simulink model "ulrich2017"  (R2023a)
settings: Solver=ode4  StartTime=0.0  StopTime=tsim  FixedStep=baseRate  RelTol=1e-6  AbsTol=1e-6
values from neighbouring files (symbols this model uses):
  Gamma1_el = 0.12    [initSpotDefaultParam.m]
  Gamma1_sh = 0.005    [initSpotDefaultParam.m]
  Gamma1_wr = 0.025    [initSpotDefaultParam.m]
  Gamma2_el = 5    [initSpotDefaultParam.m]
  Gamma2_sh = 5    [initSpotDefaultParam.m]
  Gamma2_wr = 5    [initSpotDefaultParam.m]
  Gamma3_el = 10    [initSpotDefaultParam.m]
  Gamma3_sh = 40    [initSpotDefaultParam.m]
  Gamma3_wr = 40    [initSpotDefaultParam.m]
  Gamma4_el = 0.039    [initSpotDefaultParam.m]
  Gamma4_sh = 0.015    [initSpotDefaultParam.m]
  Gamma4_wr = 0.029    [initSpotDefaultParam.m]
  Gamma5_el = 800    [initSpotDefaultParam.m]
  Gamma5_sh = 800    [initSpotDefaultParam.m]
  Gamma5_wr = 800    [initSpotDefaultParam.m]
  Gamma6_el = 0.000001    (= 1e-06)    [initSpotDefaultParam.m]
  Gamma6_sh = 0.005    [initSpotDefaultParam.m]
  Gamma6_wr = 0.02    [initSpotDefaultParam.m]
  Kd_elarm = 0.8    [initSpotDefaultParam.m]
  Kd_sharm = 1.0    (= 1)    [initSpotDefaultParam.m]
  Kd_wrarm = 0.6    [initSpotDefaultParam.m]
  Kp_elarm = 1.2    [initSpotDefaultParam.m]
  Kp_sharm = 1.5    [initSpotDefaultParam.m]
  Kp_wrarm = 2    [initSpotDefaultParam.m]
  PWMFreq = 5    [initSpotDefaultParam.m]
  Tz_lim_elarm = .1    (= 0.1)    [initSpotDefaultParam.m]
  Tz_lim_sharm = .1    (= 0.1)    [initSpotDefaultParam.m]
  Tz_lim_wrarm = .1    (= 0.1)    [initSpotDefaultParam.m]
undefined symbols (not defined in the file or in its folder): a1, a2, a3, b0, b1, b2, b3, baseRate, DiscIntNeverNeededParam, drop_states_ARM, drop_states_BLACK, drop_states_BLUE, drop_states_RED, F_Black_X_nominal, F_Black_Y_nominal, F_Blue_X_nominal, F_Blue_Y_nominal, F_red_X_nominal, F_red_Y_nominal, F_thrusters_BLACK, F_thrusters_BLUE, F_thrusters_RED, home_states_BLACK, home_states_BLUE, home_states_RED, IBLACK, IBLUE, IDIST, IEE, init_states_BLACK, init_states_BLUE, init_states_RED, IPROX, IRED, Kd_tb, Kd_tblue, Kd_tr, Kd_xb, Kd_xblue, Kd_xr, Kd_yb, Kd_yblue, Kd_yr, Kp_tb, Kp_tblue, Kp_tr, Kp_xb, Kp_xblue, Kp_xr, Kp_yb, Kp_yblue, Kp_yr, mBLACK, mBLUE, mDIST, mEE, mPROX, mRED, noise_variance_BLACK, noise_variance_BLUE ... (+24)
libraries: nvidiaSharedBlocks x9, MainLibrary x4, dspsigops x4, simulink x1
(part 7 of 11)

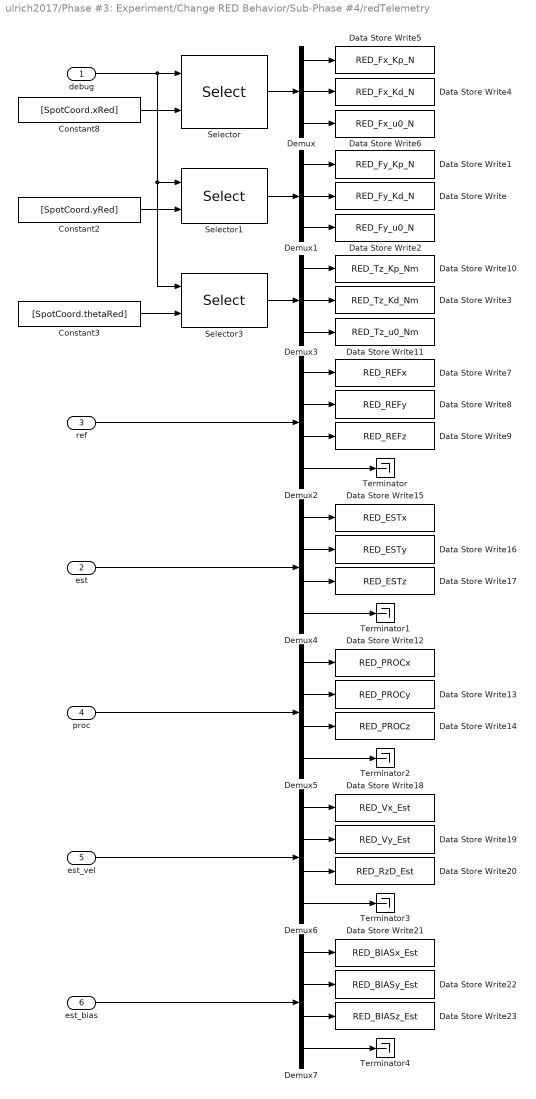
== system ulrich2017/Phase #3: Experiment/Change RED Behavior/Sub-Phase #4/redTelemetry ==
  debug : Inport
  est : Inport  Port=2
  ref : Inport  Port=3
  proc : Inport  Port=4
  est_vel : Inport  Port=5
  est_bias : Inport  Port=6
  Constant2 : Constant  Value=[SpotCoord.yRed]  VectorParams1D=off
  Constant3 : Constant  Value=[SpotCoord.thetaRed]  VectorParams1D=off
  Constant8 : Constant  Value=[SpotCoord.xRed]  VectorParams1D=off
  Data Store Write : DataStoreWrite  DataStoreName=RED_Fy_Kd_N  IndexOptions=Index vector (dialog)  Indices=1  OutputSizes=1
  Data Store Write1 : DataStoreWrite  DataStoreName=RED_Fy_Kp_N  IndexOptions=Index vector (dialog)  Indices=1  OutputSizes=1
  Data Store Write10 : DataStoreWrite  DataStoreName=RED_Tz_Kp_Nm  IndexOptions=Index vector (dialog)  Indices=1  OutputSizes=1
  Data Store Write11 : DataStoreWrite  DataStoreName=RED_Tz_u0_Nm  IndexOptions=Index vector (dialog)  Indices=1  OutputSizes=1
  Data Store Write12 : DataStoreWrite  DataStoreName=RED_PROCx  IndexOptions=Index vector (dialog)  Indices=1  OutputSizes=1
  Data Store Write13 : DataStoreWrite  DataStoreName=RED_PROCy  IndexOptions=Index vector (dialog)  Indices=1  OutputSizes=1
  Data Store Write14 : DataStoreWrite  DataStoreName=RED_PROCz  IndexOptions=Index vector (dialog)  Indices=1  OutputSizes=1
  Data Store Write15 : DataStoreWrite  DataStoreName=RED_ESTx  IndexOptions=Index vector (dialog)  Indices=1  OutputSizes=1
  Data Store Write16 : DataStoreWrite  DataStoreName=RED_ESTy  IndexOptions=Index vector (dialog)  Indices=1  OutputSizes=1
  Data Store Write17 : DataStoreWrite  DataStoreName=RED_ESTz  IndexOptions=Index vector (dialog)  Indices=1  OutputSizes=1
  Data Store Write18 : DataStoreWrite  DataStoreName=RED_Vx_Est  IndexOptions=Index vector (dialog)  Indices=1  OutputSizes=1
  Data Store Write19 : DataStoreWrite  DataStoreName=RED_Vy_Est  IndexOptions=Index vector (dialog)  Indices=1  OutputSizes=1
  Data Store Write2 : DataStoreWrite  DataStoreName=RED_Fy_u0_N  IndexOptions=Index vector (dialog)  Indices=1  OutputSizes=1
  Data Store Write20 : DataStoreWrite  DataStoreName=RED_RzD_Est  IndexOptions=Index vector (dialog)  Indices=1  OutputSizes=1
  Data Store Write21 : DataStoreWrite  DataStoreName=RED_BIASx_Est  IndexOptions=Index vector (dialog)  Indices=1  OutputSizes=1
  Data Store Write22 : DataStoreWrite  DataStoreName=RED_BIASy_Est  IndexOptions=Index vector (dialog)  Indices=1  OutputSizes=1
  Data Store Write23 : DataStoreWrite  DataStoreName=RED_BIASz_Est  IndexOptions=Index vector (dialog)  Indices=1  OutputSizes=1
  Data Store Write3 : DataStoreWrite  DataStoreName=RED_Tz_Kd_Nm  IndexOptions=Index vector (dialog)  Indices=1  OutputSizes=1
  Data Store Write4 : DataStoreWrite  DataStoreName=RED_Fx_Kd_N  IndexOptions=Index vector (dialog)  Indices=1  OutputSizes=1
  Data Store Write5 : DataStoreWrite  DataStoreName=RED_Fx_Kp_N  IndexOptions=Index vector (dialog)  Indices=1  OutputSizes=1
  Data Store Write6 : DataStoreWrite  DataStoreName=RED_Fx_u0_N  IndexOptions=Index vector (dialog)  Indices=1  OutputSizes=1
  Data Store Write7 : DataStoreWrite  DataStoreName=RED_REFx  IndexOptions=Index vector (dialog)  Indices=1  OutputSizes=1
  Data Store Write8 : DataStoreWrite  DataStoreName=RED_REFy  IndexOptions=Index vector (dialog)  Indices=1  OutputSizes=1
  Data Store Write9 : DataStoreWrite  DataStoreName=RED_REFz  IndexOptions=Index vector (dialog)  Indices=1  OutputSizes=1
  Demux : Demux  Outputs=3
  Demux1 : Demux  Outputs=3
  Demux{2,4..7} (5 alike) : Demux  Outputs=[1 1 1 9]
  Demux3 : Demux  Outputs=3
  Selector : Selector  NumberOfDimensions=2  InputPortWidth=3  IndexOptions=Select all,Index vector (port)  Indices=[1 3],1  OutputSizes=1,1
  Selector1 : Selector  NumberOfDimensions=2  InputPortWidth=3  IndexOptions=Select all,Index vector (port)  Indices=[1 3],1  OutputSizes=1,1
  Selector3 : Selector  NumberOfDimensions=2  InputPortWidth=3  IndexOptions=Select all,Index vector (port)  Indices=[1 3],1  OutputSizes=1,1
  Terminator{,1..4} (5 alike) : Terminator
  wires:
  Demux/3 -> Data Store Write6/1
  Demux/1 -> Data Store Write5/1
  Constant8/1 -> Selector/2
  Selector/1 -> Demux/1
  Demux/2 -> Data Store Write4/1
  Demux2/1 -> Data Store Write7/1
  ref/1 -> Demux2/1
  Demux2/2 -> Data Store Write8/1
  Demux2/3 -> Data Store Write9/1
  debug/1 -> Selector3/1, Selector1/1, Selector/1
  Selector1/1 -> Demux1/1
  Demux1/2 -> Data Store Write/1
  Demux1/1 -> Data Store Write1/1
  Demux1/3 -> Data Store Write2/1
  Demux3/1 -> Data Store Write10/1
  Selector3/1 -> Demux3/1
  Demux3/3 -> Data Store Write11/1
  Demux3/2 -> Data Store Write3/1
  Constant2/1 -> Selector1/2
  Constant3/1 -> Selector3/2
  Demux2/4 -> Terminator/1
  Demux4/1 -> Data Store Write15/1
  est/1 -> Demux4/1
  Demux4/2 -> Data Store Write16/1
  Demux4/3 -> Data Store Write17/1
  Demux4/4 -> Terminator1/1
  Demux5/4 -> Terminator2/1
  proc/1 -> Demux5/1
  Demux5/3 -> Data Store Write14/1
  Demux5/2 -> Data Store Write13/1
  Demux5/1 -> Data Store Write12/1
  Demux6/1 -> Data Store Write18/1
  Demux6/4 -> Terminator3/1
  est_vel/1 -> Demux6/1
  Demux6/3 -> Data Store Write20/1
  Demux6/2 -> Data Store Write19/1
  Demux7/1 -> Data Store Write21/1
  Demux7/4 -> Terminator4/1
  est_bias/1 -> Demux7/1
  Demux7/3 -> Data Store Write23/1
  Demux7/2 -> Data Store Write22/1

== system ulrich2017/Phase #4: Return Home/Change BLACK Behavior/Custom Discrete PD (Attitude)/x_dot -> x1 ==
  note: dy/dt ~= (y2-y1)/deltaT
  y(t) : Inport
  Delay1 : Delay  DelayLength=1  InitialConditionSource=Input port
      settings: InputPortMap=u0,p4
  Hold this value : Subsystem  TreatAsAtomicUnit=on
  Sum6 : Sum  Inputs=-+|
  divide by delta T : Gain  Gain=1/baseRate
  "if we went through a \"step\"" : If  IfExpression=u1 ~= 0  ShowElse=off
  dy(t)/dt : Outport  VectorParamsAs1DForOutWhenUnconnected=off
  wires:
  divide by delta T/1 -> dy(t)/dt/1
  Delay1/1 -> Sum6/1
  "if we went through a \"step\""/1 -> Hold this value/Action
  Hold this value/1(Out1) -> divide by delta T/1
  Sum6/1 -> "if we went through a \"step\""/1, Hold this value/1(In1)
  y(t)/1 -> Sum6/2, Delay1/2, Delay1/1

== system ulrich2017/Phase #4: Return Home/Change BLACK Behavior/Custom Discrete PD (X-Position)/x_dot -> x1 ==
  note: dy/dt ~= (y2-y1)/deltaT
  y(t) : Inport
  Delay1 : Delay  DelayLength=1  InitialConditionSource=Input port
      settings: InputPortMap=u0,p4
  Hold this value : Subsystem  TreatAsAtomicUnit=on
  Sum6 : Sum  Inputs=-+|
  divide by delta T : Gain  Gain=1/baseRate
  "if we went through a \"step\"" : If  IfExpression=u1 ~= 0  ShowElse=off
  dy(t)/dt : Outport  VectorParamsAs1DForOutWhenUnconnected=off
  wires:
  divide by delta T/1 -> dy(t)/dt/1
  Delay1/1 -> Sum6/1
  "if we went through a \"step\""/1 -> Hold this value/Action
  Hold this value/1(Out1) -> divide by delta T/1
  Sum6/1 -> "if we went through a \"step\""/1, Hold this value/1(In1)
  y(t)/1 -> Sum6/2, Delay1/2, Delay1/1

== system ulrich2017/Phase #4: Return Home/Change BLACK Behavior/Custom Discrete PD (Y-Position)/x_dot -> x1 ==
  note: dy/dt ~= (y2-y1)/deltaT
  y(t) : Inport
  Delay1 : Delay  DelayLength=1  InitialConditionSource=Input port
      settings: InputPortMap=u0,p4
  Hold this value : Subsystem  TreatAsAtomicUnit=on
  Sum6 : Sum  Inputs=-+|
  divide by delta T : Gain  Gain=1/baseRate
  "if we went through a \"step\"" : If  IfExpression=u1 ~= 0  ShowElse=off
  dy(t)/dt : Outport  VectorParamsAs1DForOutWhenUnconnected=off
  wires:
  divide by delta T/1 -> dy(t)/dt/1
  Delay1/1 -> Sum6/1
  "if we went through a \"step\""/1 -> Hold this value/Action
  Hold this value/1(Out1) -> divide by delta T/1
  Sum6/1 -> "if we went through a \"step\""/1, Hold this value/1(In1)
  y(t)/1 -> Sum6/2, Delay1/2, Delay1/1

== system ulrich2017/Phase #4: Return Home/Change BLUE Behavior/Custom Discrete PD (Attitude)/x_dot -> x1 ==
  note: dy/dt ~= (y2-y1)/deltaT
  y(t) : Inport
  Delay1 : Delay  DelayLength=1  InitialConditionSource=Input port
      settings: InputPortMap=u0,p4
  Hold this value : Subsystem  TreatAsAtomicUnit=on
  Sum6 : Sum  Inputs=-+|
  divide by delta T : Gain  Gain=1/baseRate
  "if we went through a \"step\"" : If  IfExpression=u1 ~= 0  ShowElse=off
  dy(t)/dt : Outport  VectorParamsAs1DForOutWhenUnconnected=off
  wires:
  divide by delta T/1 -> dy(t)/dt/1
  Delay1/1 -> Sum6/1
  "if we went through a \"step\""/1 -> Hold this value/Action
  Hold this value/1(Out1) -> divide by delta T/1
  Sum6/1 -> "if we went through a \"step\""/1, Hold this value/1(In1)
  y(t)/1 -> Sum6/2, Delay1/2, Delay1/1

== system ulrich2017/Phase #4: Return Home/Change BLUE Behavior/Custom Discrete PD (X-Position)/x_dot -> x1 ==
  note: dy/dt ~= (y2-y1)/deltaT
  y(t) : Inport
  Delay1 : Delay  DelayLength=1  InitialConditionSource=Input port
      settings: InputPortMap=u0,p4
  Hold this value : Subsystem  TreatAsAtomicUnit=on
  Sum6 : Sum  Inputs=-+|
  divide by delta T : Gain  Gain=1/baseRate
  "if we went through a \"step\"" : If  IfExpression=u1 ~= 0  ShowElse=off
  dy(t)/dt : Outport  VectorParamsAs1DForOutWhenUnconnected=off
  wires:
  divide by delta T/1 -> dy(t)/dt/1
  Delay1/1 -> Sum6/1
  "if we went through a \"step\""/1 -> Hold this value/Action
  Hold this value/1(Out1) -> divide by delta T/1
  Sum6/1 -> "if we went through a \"step\""/1, Hold this value/1(In1)
  y(t)/1 -> Sum6/2, Delay1/2, Delay1/1

== system ulrich2017/Phase #4: Return Home/Change BLUE Behavior/Custom Discrete PD (Y-Position)/x_dot -> x1 ==
  note: dy/dt ~= (y2-y1)/deltaT
  y(t) : Inport
  Delay1 : Delay  DelayLength=1  InitialConditionSource=Input port
      settings: InputPortMap=u0,p4
  Hold this value : Subsystem  TreatAsAtomicUnit=on
  Sum6 : Sum  Inputs=-+|
  divide by delta T : Gain  Gain=1/baseRate
  "if we went through a \"step\"" : If  IfExpression=u1 ~= 0  ShowElse=off
  dy(t)/dt : Outport  VectorParamsAs1DForOutWhenUnconnected=off
  wires:
  divide by delta T/1 -> dy(t)/dt/1
  Delay1/1 -> Sum6/1
  "if we went through a \"step\""/1 -> Hold this value/Action
  Hold this value/1(Out1) -> divide by delta T/1
  Sum6/1 -> "if we went through a \"step\""/1, Hold this value/1(In1)
  y(t)/1 -> Sum6/2, Delay1/2, Delay1/1

== system ulrich2017/Phase #4: Return Home/Change RED Behavior/Custom Discrete PD (Attitude)/x_dot -> x2 ==
  note: dy/dt ~= (y2-y1)/deltaT
  y(t) : Inport
  Delay1 : Delay  DelayLength=1  InitialConditionSource=Input port
      settings: InputPortMap=u0,p4
  Hold this value : Subsystem  TreatAsAtomicUnit=on
  Sum6 : Sum  Inputs=-+|
  divide by delta T : Gain  Gain=1/baseRate
  "if we went through a \"step\"" : If  IfExpression=u1 ~= 0  ShowElse=off
  dy(t)/dt : Outport  VectorParamsAs1DForOutWhenUnconnected=off
  wires:
  divide by delta T/1 -> dy(t)/dt/1
  Delay1/1 -> Sum6/1
  "if we went through a \"step\""/1 -> Hold this value/Action
  Hold this value/1(Out1) -> divide by delta T/1
  Sum6/1 -> "if we went through a \"step\""/1, Hold this value/1(In1)
  y(t)/1 -> Sum6/2, Delay1/2, Delay1/1

== system ulrich2017/Phase #4: Return Home/Change RED Behavior/Custom Discrete PD (X-Position)/x_dot -> x2 ==
  note: dy/dt ~= (y2-y1)/deltaT
  y(t) : Inport
  Delay1 : Delay  DelayLength=1  InitialConditionSource=Input port
      settings: InputPortMap=u0,p4
  Hold this value : Subsystem  TreatAsAtomicUnit=on
  Sum6 : Sum  Inputs=-+|
  divide by delta T : Gain  Gain=1/baseRate
  "if we went through a \"step\"" : If  IfExpression=u1 ~= 0  ShowElse=off
  dy(t)/dt : Outport  VectorParamsAs1DForOutWhenUnconnected=off
  wires:
  divide by delta T/1 -> dy(t)/dt/1
  Delay1/1 -> Sum6/1
  "if we went through a \"step\""/1 -> Hold this value/Action
  Hold this value/1(Out1) -> divide by delta T/1
  Sum6/1 -> "if we went through a \"step\""/1, Hold this value/1(In1)
  y(t)/1 -> Sum6/2, Delay1/2, Delay1/1

== system ulrich2017/Phase #4: Return Home/Change RED Behavior/Custom Discrete PD (Y-Position)/x_dot -> x2 ==
  note: dy/dt ~= (y2-y1)/deltaT
  y(t) : Inport
  Delay1 : Delay  DelayLength=1  InitialConditionSource=Input port
      settings: InputPortMap=u0,p4
  Hold this value : Subsystem  TreatAsAtomicUnit=on
  Sum6 : Sum  Inputs=-+|
  divide by delta T : Gain  Gain=1/baseRate
  "if we went through a \"step\"" : If  IfExpression=u1 ~= 0  ShowElse=off
  dy(t)/dt : Outport  VectorParamsAs1DForOutWhenUnconnected=off
  wires:
  divide by delta T/1 -> dy(t)/dt/1
  Delay1/1 -> Sum6/1
  "if we went through a \"step\""/1 -> Hold this value/Action
  Hold this value/1(Out1) -> divide by delta T/1
  Sum6/1 -> "if we went through a \"step\""/1, Hold this value/1(In1)
  y(t)/1 -> Sum6/2, Delay1/2, Delay1/1

== system ulrich2017/Phase #4: Return Home/Change RED Behavior/RED+ARM/Passthrough for Experiment ==
  q1_desired : Inport
  q2_desired : Inport  Port=2
  q3_desired : Inport  Port=3
  Action Port : ActionPort  ActionPortLabel=else
  q1_command : Outport
  q2_command : Outport  Port=2
  q3_command : Outport  Port=3
  wires:
  q3_desired/1 -> q3_command/1
  q1_desired/1 -> q1_command/1
  q2_desired/1 -> q2_command/1

== system ulrich2017/Phase #4: Return Home/Change RED Behavior/RED+ARM/Simulated Position Controller ==
  q1_desired : Inport
  q2_desired : Inport  Port=2
  q3_desired : Inport  Port=3
  Action Port : ActionPort  ActionPortLabel=if(u1 == 1)
  Custom Discrete PD (Elbow) : Subsystem
  Custom Discrete PD (Shoulder) : Subsystem
  Custom Discrete PD (Wrist) : Subsystem
  Data Store Read : DataStoreRead  DataStoreName=RED_Rz_Shoulder  IndexOptions=Index vector (dialog)  Indices=1  OutputSizes=1
  Data Store Read5 : DataStoreRead  DataStoreName=RED_Rz_Elbow  IndexOptions=Index vector (dialog)  Indices=1  OutputSizes=1
  Data Store Read6 : DataStoreRead  DataStoreName=RED_Rz_Wrist  IndexOptions=Index vector (dialog)  Indices=1  OutputSizes=1
  Saturation : Saturate  UpperLimit=Tz_lim_sharm  LowerLimit=-Tz_lim_sharm
  Saturation1 : Saturate  UpperLimit=Tz_lim_elarm  LowerLimit=-Tz_lim_elarm
  Saturation3 : Saturate  UpperLimit=Tz_lim_wrarm  LowerLimit=-Tz_lim_wrarm
  Subtract2 : Sum  Inputs=+-
  Subtract3 : Sum  Inputs=+-
  Subtract4 : Sum  Inputs=+-
  q1_command : Outport
  q2_command : Outport  Port=2
  q3_command : Outport  Port=3
  wires:
  Saturation3/1 -> q3_command/1
  Subtract4/1 -> Custom Discrete PD (Wrist)/1(ey)
  Custom Discrete PD (Shoulder)/1(Fx) -> Saturation/1
  Custom Discrete PD (Elbow)/1(Fy) -> Saturation1/1
  Saturation/1 -> q1_command/1
  Subtract2/1 -> Custom Discrete PD (Shoulder)/1(ex)
  Saturation1/1 -> q2_command/1
  Custom Discrete PD (Wrist)/1(Fy) -> Saturation3/1
  Subtract3/1 -> Custom Discrete PD (Elbow)/1(ey)
  Data Store Read/1 -> Subtract2/2
  Data Store Read5/1 -> Subtract3/2
  Data Store Read6/1 -> Subtract4/2
  q1_desired/1 -> Subtract2/1
  q2_desired/1 -> Subtract3/1
  q3_desired/1 -> Subtract4/1

== system ulrich2017/Phase #5: Hold Home/Change BLACK Behavior/Custom Discrete PD (Attitude)/x_dot -> x1 ==
  note: dy/dt ~= (y2-y1)/deltaT
  y(t) : Inport
  Delay1 : Delay  DelayLength=1  InitialConditionSource=Input port
      settings: InputPortMap=u0,p4
  Hold this value : Subsystem  TreatAsAtomicUnit=on
  Sum6 : Sum  Inputs=-+|
  divide by delta T : Gain  Gain=1/baseRate
  "if we went through a \"step\"" : If  IfExpression=u1 ~= 0  ShowElse=off
  dy(t)/dt : Outport  VectorParamsAs1DForOutWhenUnconnected=off
  wires:
  divide by delta T/1 -> dy(t)/dt/1
  Delay1/1 -> Sum6/1
  "if we went through a \"step\""/1 -> Hold this value/Action
  Hold this value/1(Out1) -> divide by delta T/1
  Sum6/1 -> "if we went through a \"step\""/1, Hold this value/1(In1)
  y(t)/1 -> Sum6/2, Delay1/2, Delay1/1

== system ulrich2017/Phase #5: Hold Home/Change BLACK Behavior/Custom Discrete PD (X-Position)/x_dot -> x1 ==
  note: dy/dt ~= (y2-y1)/deltaT
  y(t) : Inport
  Delay1 : Delay  DelayLength=1  InitialConditionSource=Input port
      settings: InputPortMap=u0,p4
  Hold this value : Subsystem  TreatAsAtomicUnit=on
  Sum6 : Sum  Inputs=-+|
  divide by delta T : Gain  Gain=1/baseRate
  "if we went through a \"step\"" : If  IfExpression=u1 ~= 0  ShowElse=off
  dy(t)/dt : Outport  VectorParamsAs1DForOutWhenUnconnected=off
  wires:
  divide by delta T/1 -> dy(t)/dt/1
  Delay1/1 -> Sum6/1
  "if we went through a \"step\""/1 -> Hold this value/Action
  Hold this value/1(Out1) -> divide by delta T/1
  Sum6/1 -> "if we went through a \"step\""/1, Hold this value/1(In1)
  y(t)/1 -> Sum6/2, Delay1/2, Delay1/1

== system ulrich2017/Phase #5: Hold Home/Change BLACK Behavior/Custom Discrete PD (Y-Position)/x_dot -> x1 ==
  note: dy/dt ~= (y2-y1)/deltaT
  y(t) : Inport
  Delay1 : Delay  DelayLength=1  InitialConditionSource=Input port
      settings: InputPortMap=u0,p4
  Hold this value : Subsystem  TreatAsAtomicUnit=on
  Sum6 : Sum  Inputs=-+|
  divide by delta T : Gain  Gain=1/baseRate
  "if we went through a \"step\"" : If  IfExpression=u1 ~= 0  ShowElse=off
  dy(t)/dt : Outport  VectorParamsAs1DForOutWhenUnconnected=off
  wires:
  divide by delta T/1 -> dy(t)/dt/1
  Delay1/1 -> Sum6/1
  "if we went through a \"step\""/1 -> Hold this value/Action
  Hold this value/1(Out1) -> divide by delta T/1
  Sum6/1 -> "if we went through a \"step\""/1, Hold this value/1(In1)
  y(t)/1 -> Sum6/2, Delay1/2, Delay1/1

== system ulrich2017/Phase #5: Hold Home/Change BLUE Behavior/Custom Discrete PD (Attitude)/x_dot -> x1 ==
  note: dy/dt ~= (y2-y1)/deltaT
  y(t) : Inport
  Delay1 : Delay  DelayLength=1  InitialConditionSource=Input port
      settings: InputPortMap=u0,p4
  Hold this value : Subsystem  TreatAsAtomicUnit=on
  Sum6 : Sum  Inputs=-+|
  divide by delta T : Gain  Gain=1/baseRate
  "if we went through a \"step\"" : If  IfExpression=u1 ~= 0  ShowElse=off
  dy(t)/dt : Outport  VectorParamsAs1DForOutWhenUnconnected=off
  wires:
  divide by delta T/1 -> dy(t)/dt/1
  Delay1/1 -> Sum6/1
  "if we went through a \"step\""/1 -> Hold this value/Action
  Hold this value/1(Out1) -> divide by delta T/1
  Sum6/1 -> "if we went through a \"step\""/1, Hold this value/1(In1)
  y(t)/1 -> Sum6/2, Delay1/2, Delay1/1

== system ulrich2017/Phase #5: Hold Home/Change BLUE Behavior/Custom Discrete PD (X-Position)/x_dot -> x1 ==
  note: dy/dt ~= (y2-y1)/deltaT
  y(t) : Inport
  Delay1 : Delay  DelayLength=1  InitialConditionSource=Input port
      settings: InputPortMap=u0,p4
  Hold this value : Subsystem  TreatAsAtomicUnit=on
  Sum6 : Sum  Inputs=-+|
  divide by delta T : Gain  Gain=1/baseRate
  "if we went through a \"step\"" : If  IfExpression=u1 ~= 0  ShowElse=off
  dy(t)/dt : Outport  VectorParamsAs1DForOutWhenUnconnected=off
  wires:
  divide by delta T/1 -> dy(t)/dt/1
  Delay1/1 -> Sum6/1
  "if we went through a \"step\""/1 -> Hold this value/Action
  Hold this value/1(Out1) -> divide by delta T/1
  Sum6/1 -> "if we went through a \"step\""/1, Hold this value/1(In1)
  y(t)/1 -> Sum6/2, Delay1/2, Delay1/1

== system ulrich2017/Phase #5: Hold Home/Change BLUE Behavior/Custom Discrete PD (Y-Position)/x_dot -> x1 ==
  note: dy/dt ~= (y2-y1)/deltaT
  y(t) : Inport
  Delay1 : Delay  DelayLength=1  InitialConditionSource=Input port
      settings: InputPortMap=u0,p4
  Hold this value : Subsystem  TreatAsAtomicUnit=on
  Sum6 : Sum  Inputs=-+|
  divide by delta T : Gain  Gain=1/baseRate
  "if we went through a \"step\"" : If  IfExpression=u1 ~= 0  ShowElse=off
  dy(t)/dt : Outport  VectorParamsAs1DForOutWhenUnconnected=off
  wires:
  divide by delta T/1 -> dy(t)/dt/1
  Delay1/1 -> Sum6/1
  "if we went through a \"step\""/1 -> Hold this value/Action
  Hold this value/1(Out1) -> divide by delta T/1
  Sum6/1 -> "if we went through a \"step\""/1, Hold this value/1(In1)
  y(t)/1 -> Sum6/2, Delay1/2, Delay1/1

== system ulrich2017/Phase #5: Hold Home/Change RED Behavior/Custom Discrete PD (Attitude)/x_dot -> x2 ==
  note: dy/dt ~= (y2-y1)/deltaT
  y(t) : Inport
  Delay1 : Delay  DelayLength=1  InitialConditionSource=Input port
      settings: InputPortMap=u0,p4
  Hold this value : Subsystem  TreatAsAtomicUnit=on
  Sum6 : Sum  Inputs=-+|
  divide by delta T : Gain  Gain=1/baseRate
  "if we went through a \"step\"" : If  IfExpression=u1 ~= 0  ShowElse=off
  dy(t)/dt : Outport  VectorParamsAs1DForOutWhenUnconnected=off
  wires:
  divide by delta T/1 -> dy(t)/dt/1
  Delay1/1 -> Sum6/1
  "if we went through a \"step\""/1 -> Hold this value/Action
  Hold this value/1(Out1) -> divide by delta T/1
  Sum6/1 -> "if we went through a \"step\""/1, Hold this value/1(In1)
  y(t)/1 -> Sum6/2, Delay1/2, Delay1/1

== system ulrich2017/Phase #5: Hold Home/Change RED Behavior/Custom Discrete PD (X-Position)/x_dot -> x2 ==
  note: dy/dt ~= (y2-y1)/deltaT
  y(t) : Inport
  Delay1 : Delay  DelayLength=1  InitialConditionSource=Input port
      settings: InputPortMap=u0,p4
  Hold this value : Subsystem  TreatAsAtomicUnit=on
  Sum6 : Sum  Inputs=-+|
  divide by delta T : Gain  Gain=1/baseRate
  "if we went through a \"step\"" : If  IfExpression=u1 ~= 0  ShowElse=off
  dy(t)/dt : Outport  VectorParamsAs1DForOutWhenUnconnected=off
  wires:
  divide by delta T/1 -> dy(t)/dt/1
  Delay1/1 -> Sum6/1
  "if we went through a \"step\""/1 -> Hold this value/Action
  Hold this value/1(Out1) -> divide by delta T/1
  Sum6/1 -> "if we went through a \"step\""/1, Hold this value/1(In1)
  y(t)/1 -> Sum6/2, Delay1/2, Delay1/1

== system ulrich2017/Phase #5: Hold Home/Change RED Behavior/Custom Discrete PD (Y-Position)/x_dot -> x2 ==
  note: dy/dt ~= (y2-y1)/deltaT
  y(t) : Inport
  Delay1 : Delay  DelayLength=1  InitialConditionSource=Input port
      settings: InputPortMap=u0,p4
  Hold this value : Subsystem  TreatAsAtomicUnit=on
  Sum6 : Sum  Inputs=-+|
  divide by delta T : Gain  Gain=1/baseRate
  "if we went through a \"step\"" : If  IfExpression=u1 ~= 0  ShowElse=off
  dy(t)/dt : Outport  VectorParamsAs1DForOutWhenUnconnected=off
  wires:
  divide by delta T/1 -> dy(t)/dt/1
  Delay1/1 -> Sum6/1
  "if we went through a \"step\""/1 -> Hold this value/Action
  Hold this value/1(Out1) -> divide by delta T/1
  Sum6/1 -> "if we went through a \"step\""/1, Hold this value/1(In1)
  y(t)/1 -> Sum6/2, Delay1/2, Delay1/1

== system ulrich2017/Phase #5: Hold Home/Change RED Behavior/RED+ARM/Passthrough for Experiment ==
  q1_desired : Inport
  q2_desired : Inport  Port=2
  q3_desired : Inport  Port=3
  Action Port : ActionPort  ActionPortLabel=else
  q1_command : Outport
  q2_command : Outport  Port=2
  q3_command : Outport  Port=3
  wires:
  q3_desired/1 -> q3_command/1
  q1_desired/1 -> q1_command/1
  q2_desired/1 -> q2_command/1

== system ulrich2017/Phase #5: Hold Home/Change RED Behavior/RED+ARM/Simulated Position Controller ==
  q1_desired : Inport
  q2_desired : Inport  Port=2
  q3_desired : Inport  Port=3
  Action Port : ActionPort  ActionPortLabel=if(u1 == 1)
  Custom Discrete PD (Elbow) : Subsystem
  Custom Discrete PD (Shoulder) : Subsystem
  Custom Discrete PD (Wrist) : Subsystem
  Data Store Read : DataStoreRead  DataStoreName=RED_Rz_Shoulder  IndexOptions=Index vector (dialog)  Indices=1  OutputSizes=1
  Data Store Read5 : DataStoreRead  DataStoreName=RED_Rz_Elbow  IndexOptions=Index vector (dialog)  Indices=1  OutputSizes=1
  Data Store Read6 : DataStoreRead  DataStoreName=RED_Rz_Wrist  IndexOptions=Index vector (dialog)  Indices=1  OutputSizes=1
  Saturation : Saturate  UpperLimit=Tz_lim_sharm  LowerLimit=-Tz_lim_sharm
  Saturation1 : Saturate  UpperLimit=Tz_lim_elarm  LowerLimit=-Tz_lim_elarm
  Saturation3 : Saturate  UpperLimit=Tz_lim_wrarm  LowerLimit=-Tz_lim_wrarm
  Subtract2 : Sum  Inputs=+-
  Subtract3 : Sum  Inputs=+-
  Subtract4 : Sum  Inputs=+-
  q1_command : Outport
  q2_command : Outport  Port=2
  q3_command : Outport  Port=3
  wires:
  Saturation3/1 -> q3_command/1
  Subtract4/1 -> Custom Discrete PD (Wrist)/1(ey)
  Custom Discrete PD (Shoulder)/1(Fx) -> Saturation/1
  Custom Discrete PD (Elbow)/1(Fy) -> Saturation1/1
  Saturation/1 -> q1_command/1
  Subtract2/1 -> Custom Discrete PD (Shoulder)/1(ex)
  Saturation1/1 -> q2_command/1
  Custom Discrete PD (Wrist)/1(Fy) -> Saturation3/1
  Subtract3/1 -> Custom Discrete PD (Elbow)/1(ey)
  Data Store Read/1 -> Subtract2/2
  Data Store Read5/1 -> Subtract3/2
  Data Store Read6/1 -> Subtract4/2
  q1_desired/1 -> Subtract2/1
  q2_desired/1 -> Subtract3/1
  q3_desired/1 -> Subtract4/1

== system ulrich2017/PhaseSpace Camera Code/Use Hardware to Obtain States/Adjust Time/Enabled Subsystem ==
  In1 : Inport
  Enable : EnablePort
  Memory : Memory
  Out1 : Outport
  wires:
  Memory/1 -> Out1/1
  In1/1 -> Memory/1

== system ulrich2017/PhaseSpace Camera Code/Use Hardware to Obtain States/Adjust Time/Enabled Subsystem1 ==
  In2 : Inport
  In1 : Inport  Port=2
  Enable : EnablePort
  Subtract : Sum  Inputs=+-
  Out1 : Outport
  wires:
  Subtract/1 -> Out1/1
  In1/1 -> Subtract/1
  In2/1 -> Subtract/2

== system ulrich2017/PhaseSpace Camera Code/Use Hardware to Obtain States/x_dot -> x1/Hold this value ==
  In1 : Inport
  Action Port : ActionPort  ActionPortLabel=if(u1 ~= 0)
  Out1 : Outport  VectorParamsAs1DForOutWhenUnconnected=off
  wires:
  In1/1 -> Out1/1

== system ulrich2017/PhaseSpace Camera Code/Use Hardware to Obtain States/x_dot -> x10/Hold this value ==
  In1 : Inport
  Action Port : ActionPort  ActionPortLabel=if(u1 ~= 0)
  Out1 : Outport  VectorParamsAs1DForOutWhenUnconnected=off
  wires:
  In1/1 -> Out1/1

== system ulrich2017/PhaseSpace Camera Code/Use Hardware to Obtain States/x_dot -> x11/Hold this value ==
  In1 : Inport
  Action Port : ActionPort  ActionPortLabel=if(u1 ~= 0)
  Out1 : Outport  VectorParamsAs1DForOutWhenUnconnected=off
  wires:
  In1/1 -> Out1/1

== system ulrich2017/PhaseSpace Camera Code/Use Hardware to Obtain States/x_dot -> x12/Hold this value ==
  In1 : Inport
  Action Port : ActionPort  ActionPortLabel=if(u1 ~= 0)
  Out1 : Outport  VectorParamsAs1DForOutWhenUnconnected=off
  wires:
  In1/1 -> Out1/1

== system ulrich2017/PhaseSpace Camera Code/Use Hardware to Obtain States/x_dot -> x13/Hold this value ==
  In1 : Inport
  Action Port : ActionPort  ActionPortLabel=if(u1 ~= 0)
  Out1 : Outport  VectorParamsAs1DForOutWhenUnconnected=off
  wires:
  In1/1 -> Out1/1

== system ulrich2017/PhaseSpace Camera Code/Use Hardware to Obtain States/x_dot -> x14/Hold this value ==
  In1 : Inport
  Action Port : ActionPort  ActionPortLabel=if(u1 ~= 0)
  Out1 : Outport  VectorParamsAs1DForOutWhenUnconnected=off
  wires:
  In1/1 -> Out1/1

== system ulrich2017/PhaseSpace Camera Code/Use Hardware to Obtain States/x_dot -> x15/Hold this value ==
  In1 : Inport
  Action Port : ActionPort  ActionPortLabel=if(u1 ~= 0)
  Out1 : Outport  VectorParamsAs1DForOutWhenUnconnected=off
  wires:
  In1/1 -> Out1/1

== system ulrich2017/PhaseSpace Camera Code/Use Hardware to Obtain States/x_dot -> x16/Hold this value ==
  In1 : Inport
  Action Port : ActionPort  ActionPortLabel=if(u1 ~= 0)
  Out1 : Outport  VectorParamsAs1DForOutWhenUnconnected=off
  wires:
  In1/1 -> Out1/1

== system ulrich2017/PhaseSpace Camera Code/Use Hardware to Obtain States/x_dot -> x17/Hold this value ==
  In1 : Inport
  Action Port : ActionPort  ActionPortLabel=if(u1 ~= 0)
  Out1 : Outport  VectorParamsAs1DForOutWhenUnconnected=off
  wires:
  In1/1 -> Out1/1

== system ulrich2017/PhaseSpace Camera Code/Use Hardware to Obtain States/x_dot -> x18/Hold this value ==
  In1 : Inport
  Action Port : ActionPort  ActionPortLabel=if(u1 ~= 0)
  Out1 : Outport  VectorParamsAs1DForOutWhenUnconnected=off
  wires:
  In1/1 -> Out1/1

== system ulrich2017/PhaseSpace Camera Code/Use Hardware to Obtain States/x_dot -> x2/Hold this value ==
  In1 : Inport
  Action Port : ActionPort  ActionPortLabel=if(u1 ~= 0)
  Out1 : Outport  VectorParamsAs1DForOutWhenUnconnected=off
  wires:
  In1/1 -> Out1/1

== system ulrich2017/PhaseSpace Camera Code/Use Hardware to Obtain States/x_dot -> x3/Hold this value ==
  In1 : Inport
  Action Port : ActionPort  ActionPortLabel=if(u1 ~= 0)
  Out1 : Outport  VectorParamsAs1DForOutWhenUnconnected=off
  wires:
  In1/1 -> Out1/1

== system ulrich2017/PhaseSpace Camera Code/Use Hardware to Obtain States/x_dot -> x4/Hold this value ==
  In1 : Inport
  Action Port : ActionPort  ActionPortLabel=if(u1 ~= 0)
  Out1 : Outport  VectorParamsAs1DForOutWhenUnconnected=off
  wires:
  In1/1 -> Out1/1

== system ulrich2017/PhaseSpace Camera Code/Use Hardware to Obtain States/x_dot -> x5/Hold this value ==
  In1 : Inport
  Action Port : ActionPort  ActionPortLabel=if(u1 ~= 0)
  Out1 : Outport  VectorParamsAs1DForOutWhenUnconnected=off
  wires:
  In1/1 -> Out1/1

== system ulrich2017/PhaseSpace Camera Code/Use Hardware to Obtain States/x_dot -> x6/Hold this value ==
  In1 : Inport
  Action Port : ActionPort  ActionPortLabel=if(u1 ~= 0)
  Out1 : Outport  VectorParamsAs1DForOutWhenUnconnected=off
  wires:
  In1/1 -> Out1/1

== system ulrich2017/PhaseSpace Camera Code/Use Hardware to Obtain States/x_dot -> x7/Hold this value ==
  In1 : Inport
  Action Port : ActionPort  ActionPortLabel=if(u1 ~= 0)
  Out1 : Outport  VectorParamsAs1DForOutWhenUnconnected=off
  wires:
  In1/1 -> Out1/1

== system ulrich2017/PhaseSpace Camera Code/Use Hardware to Obtain States/x_dot -> x8/Hold this value ==
  In1 : Inport
  Action Port : ActionPort  ActionPortLabel=if(u1 ~= 0)
  Out1 : Outport  VectorParamsAs1DForOutWhenUnconnected=off
  wires:
  In1/1 -> Out1/1

== system ulrich2017/PhaseSpace Camera Code/Use Hardware to Obtain States/x_dot -> x9/Hold this value ==
  In1 : Inport
  Action Port : ActionPort  ActionPortLabel=if(u1 ~= 0)
  Out1 : Outport  VectorParamsAs1DForOutWhenUnconnected=off
  wires:
  In1/1 -> Out1/1

== system ulrich2017/Simulate Plant Dynamics/BLACK Dynamics/x_dot -> x1/Hold this value ==
  In1 : Inport
  Action Port : ActionPort  ActionPortLabel=if(u1 ~= 0)
  Out1 : Outport  VectorParamsAs1DForOutWhenUnconnected=off
  wires:
  In1/1 -> Out1/1

== system ulrich2017/Simulate Plant Dynamics/BLACK Dynamics/x_dot -> x2/Hold this value ==
  In1 : Inport
  Action Port : ActionPort  ActionPortLabel=if(u1 ~= 0)
  Out1 : Outport  VectorParamsAs1DForOutWhenUnconnected=off
  wires:
  In1/1 -> Out1/1

== system ulrich2017/Simulate Plant Dynamics/BLACK Dynamics/x_dot -> x3/Hold this value ==
  In1 : Inport
  Action Port : ActionPort  ActionPortLabel=if(u1 ~= 0)
  Out1 : Outport  VectorParamsAs1DForOutWhenUnconnected=off
  wires:
  In1/1 -> Out1/1

== system ulrich2017/Simulate Plant Dynamics/BLACK Dynamics/x_dot -> x4/Hold this value ==
  In1 : Inport
  Action Port : ActionPort  ActionPortLabel=if(u1 ~= 0)
  Out1 : Outport  VectorParamsAs1DForOutWhenUnconnected=off
  wires:
  In1/1 -> Out1/1

== system ulrich2017/Simulate Plant Dynamics/BLACK Dynamics/x_dot -> x5/Hold this value ==
  In1 : Inport
  Action Port : ActionPort  ActionPortLabel=if(u1 ~= 0)
  Out1 : Outport  VectorParamsAs1DForOutWhenUnconnected=off
  wires:
  In1/1 -> Out1/1

== system ulrich2017/Simulate Plant Dynamics/BLACK Dynamics/x_dot -> x7/Hold this value ==
  In1 : Inport
  Action Port : ActionPort  ActionPortLabel=if(u1 ~= 0)
  Out1 : Outport  VectorParamsAs1DForOutWhenUnconnected=off
  wires:
  In1/1 -> Out1/1

== system ulrich2017/Simulate Plant Dynamics/BLUE Dynamics/x_dot -> x1/Hold this value ==
  In1 : Inport
  Action Port : ActionPort  ActionPortLabel=if(u1 ~= 0)
  Out1 : Outport  VectorParamsAs1DForOutWhenUnconnected=off
  wires:
  In1/1 -> Out1/1

== system ulrich2017/Simulate Plant Dynamics/BLUE Dynamics/x_dot -> x2/Hold this value ==
  In1 : Inport
  Action Port : ActionPort  ActionPortLabel=if(u1 ~= 0)
  Out1 : Outport  VectorParamsAs1DForOutWhenUnconnected=off
  wires:
  In1/1 -> Out1/1

== system ulrich2017/Simulate Plant Dynamics/BLUE Dynamics/x_dot -> x3/Hold this value ==
  In1 : Inport
  Action Port : ActionPort  ActionPortLabel=if(u1 ~= 0)
  Out1 : Outport  VectorParamsAs1DForOutWhenUnconnected=off
  wires:
  In1/1 -> Out1/1

== system ulrich2017/Simulate Plant Dynamics/BLUE Dynamics/x_dot -> x4/Hold this value ==
  In1 : Inport
  Action Port : ActionPort  ActionPortLabel=if(u1 ~= 0)
  Out1 : Outport  VectorParamsAs1DForOutWhenUnconnected=off
  wires:
  In1/1 -> Out1/1

== system ulrich2017/Simulate Plant Dynamics/BLUE Dynamics/x_dot -> x5/Hold this value ==
  In1 : Inport
  Action Port : ActionPort  ActionPortLabel=if(u1 ~= 0)
  Out1 : Outport  VectorParamsAs1DForOutWhenUnconnected=off
  wires:
  In1/1 -> Out1/1

== system ulrich2017/Simulate Plant Dynamics/BLUE Dynamics/x_dot -> x7/Hold this value ==
  In1 : Inport
  Action Port : ActionPort  ActionPortLabel=if(u1 ~= 0)
  Out1 : Outport  VectorParamsAs1DForOutWhenUnconnected=off
  wires:
  In1/1 -> Out1/1

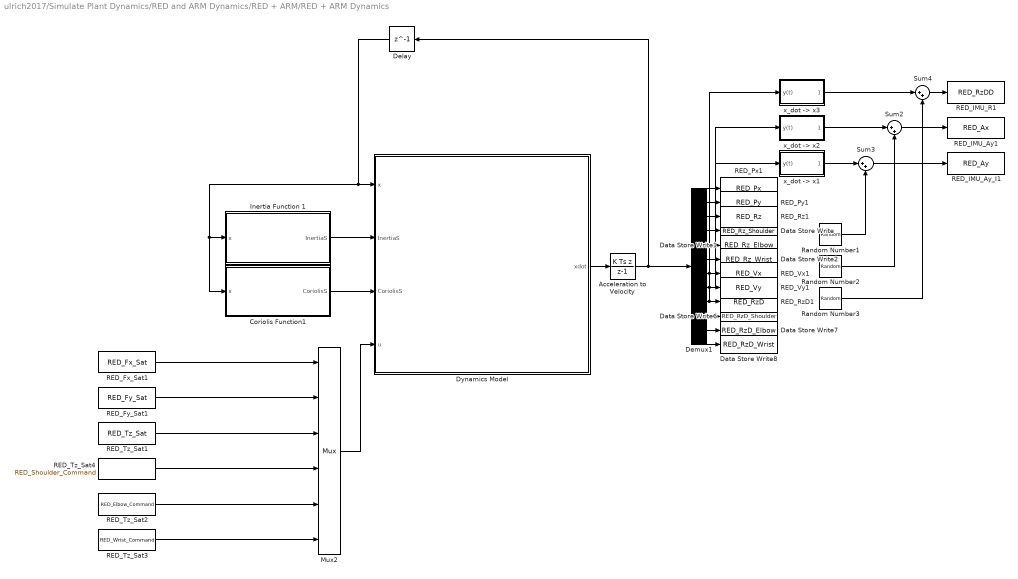
== system ulrich2017/Simulate Plant Dynamics/RED and ARM Dynamics/RED + ARM/RED + ARM Dynamics ==
  Acceleration to Velocity : DiscreteIntegrator  IntegratorMethod=Integration: Backward Euler  InitialCondition=[drop_states_RED,drop_states_ARM,0,0,0,0,0,0]  SampleTime=-1  ICPrevOutput=DiscIntNeverNeededParam  ICPrevScaledInput=DiscIntNeverNeededParam
  Coriolis Function1 : MATLAB Function  TreatAsAtomicUnit=on
  Data Store Write : DataStoreWrite  DataStoreName=RED_Rz_Shoulder  IndexOptions=Index vector (dialog)  Indices=1  OutputSizes=1
  Data Store Write1 : DataStoreWrite  DataStoreName=RED_Rz_Elbow  IndexOptions=Index vector (dialog)  Indices=1  OutputSizes=1
  Data Store Write2 : DataStoreWrite  DataStoreName=RED_Rz_Wrist  IndexOptions=Index vector (dialog)  Indices=1  OutputSizes=1
  Data Store Write6 : DataStoreWrite  DataStoreName=RED_RzD_Shoulder  IndexOptions=Index vector (dialog)  Indices=1  OutputSizes=1
  Data Store Write7 : DataStoreWrite  DataStoreName=RED_RzD_Elbow  IndexOptions=Index vector (dialog)  Indices=1  OutputSizes=1
  Data Store Write8 : DataStoreWrite  DataStoreName=RED_RzD_Wrist  IndexOptions=Index vector (dialog)  Indices=1  OutputSizes=1
  Delay : Delay  DelayLength=1
  Demux1 : Demux  Outputs=12
  Dynamics Model : MATLAB Function  TreatAsAtomicUnit=on
  Inertia Function 1 : MATLAB Function  TreatAsAtomicUnit=on
  Mux2 : Mux  Inputs=6
  RED_Fx_Sat1 : DataStoreRead  DataStoreName=RED_Fx_Sat  IndexOptions=Index vector (dialog)  Indices=1  OutputSizes=1
  RED_Fy_Sat1 : DataStoreRead  DataStoreName=RED_Fy_Sat  IndexOptions=Index vector (dialog)  Indices=1  OutputSizes=1
  RED_IMU_Ay1 : DataStoreWrite  DataStoreName=RED_Ax  IndexOptions=Index vector (dialog)  Indices=1  OutputSizes=1
  RED_IMU_Ay_I1 : DataStoreWrite  DataStoreName=RED_Ay  IndexOptions=Index vector (dialog)  Indices=1  OutputSizes=1
  RED_IMU_R1 : DataStoreWrite  DataStoreName=RED_RzDD  IndexOptions=Index vector (dialog)  Indices=1  OutputSizes=1
  RED_Px1 : DataStoreWrite  DataStoreName=RED_Px  IndexOptions=Index vector (dialog)  Indices=1  OutputSizes=1
  RED_Py1 : DataStoreWrite  DataStoreName=RED_Py  IndexOptions=Index vector (dialog)  Indices=1  OutputSizes=1
  RED_Rz1 : DataStoreWrite  DataStoreName=RED_Rz  IndexOptions=Index vector (dialog)  Indices=1  OutputSizes=1
  RED_RzD1 : DataStoreWrite  DataStoreName=RED_RzD  IndexOptions=Index vector (dialog)  Indices=1  OutputSizes=1
  RED_Tz_Sat1 : DataStoreRead  DataStoreName=RED_Tz_Sat  IndexOptions=Index vector (dialog)  Indices=1  OutputSizes=1
  RED_Tz_Sat2 : DataStoreRead  DataStoreName=RED_Elbow_Command  IndexOptions=Index vector (dialog)  Indices=1  OutputSizes=1
  RED_Tz_Sat3 : DataStoreRead  DataStoreName=RED_Wrist_Command  IndexOptions=Index vector (dialog)  Indices=1  OutputSizes=1
  RED_Tz_Sat4 : DataStoreRead  DataStoreName=RED_Shoulder_Command  IndexOptions=Index vector (dialog)  Indices=1  OutputSizes=1
  RED_Vx1 : DataStoreWrite  DataStoreName=RED_Vx  IndexOptions=Index vector (dialog)  Indices=1  OutputSizes=1
  RED_Vy1 : DataStoreWrite  DataStoreName=RED_Vy  IndexOptions=Index vector (dialog)  Indices=1  OutputSizes=1
  Random Number1 : RandomNumber  Variance=0
  Random Number2 : RandomNumber  Variance=0
  Random Number3 : RandomNumber  Variance=0
  Sum2 : Sum  Inputs=|++
  Sum3 : Sum  Inputs=|++
  Sum4 : Sum  Inputs=|++
  "x_dot -> x1" : Subsystem
  "x_dot -> x2" : Subsystem
  "x_dot -> x3" : Subsystem
  wires:
  Demux1/2 -> RED_Py1/1
  Random Number1/1 -> Sum3/2
  Random Number2/1 -> Sum2/2
  Demux1/3 -> RED_Rz1/1
  Demux1/9 -> "x_dot -> x3"/1(y(t)), RED_RzD1/1
  RED_Tz_Sat1/1 -> Mux2/3
  Delay/1 -> Dynamics Model/1(x), Coriolis Function1/1(x), Inertia Function 1/1(x)
  RED_Fx_Sat1/1 -> Mux2/1
  "x_dot -> x1"/1(dy(t)/dt) -> Sum3/1
  Demux1/8 -> "x_dot -> x1"/1(y(t)), RED_Vy1/1
  Demux1/1 -> RED_Px1/1
  "x_dot -> x2"/1(dy(t)/dt) -> Sum2/1
  Random Number3/1 -> Sum4/2
  Mux2/1 -> Dynamics Model/4(u)
  Demux1/7 -> "x_dot -> x2"/1(y(t)), RED_Vx1/1
  Demux1/12 -> Data Store Write8/1
  Inertia Function 1/1(InertiaS) -> Dynamics Model/2(InertiaS)
  Demux1/11 -> Data Store Write7/1
  Sum2/1 -> RED_IMU_Ay1/1
  Sum4/1 -> RED_IMU_R1/1
  Acceleration to Velocity/1 -> Delay/1, Demux1/1
  Dynamics Model/1(xdot) -> Acceleration to Velocity/1
  Demux1/10 -> Data Store Write6/1
  Demux1/5 -> Data Store Write1/1
  Coriolis Function1/1(CoriolisS) -> Dynamics Model/3(CoriolisS)
  Demux1/6 -> Data Store Write2/1
  Sum3/1 -> RED_IMU_Ay_I1/1
  Demux1/4 -> Data Store Write/1
  RED_Fy_Sat1/1 -> Mux2/2
  "x_dot -> x3"/1(dy(t)/dt) -> Sum4/1
  RED_Tz_Sat4/1 -> Mux2/4
  RED_Tz_Sat2/1 -> Mux2/5
  RED_Tz_Sat3/1 -> Mux2/6

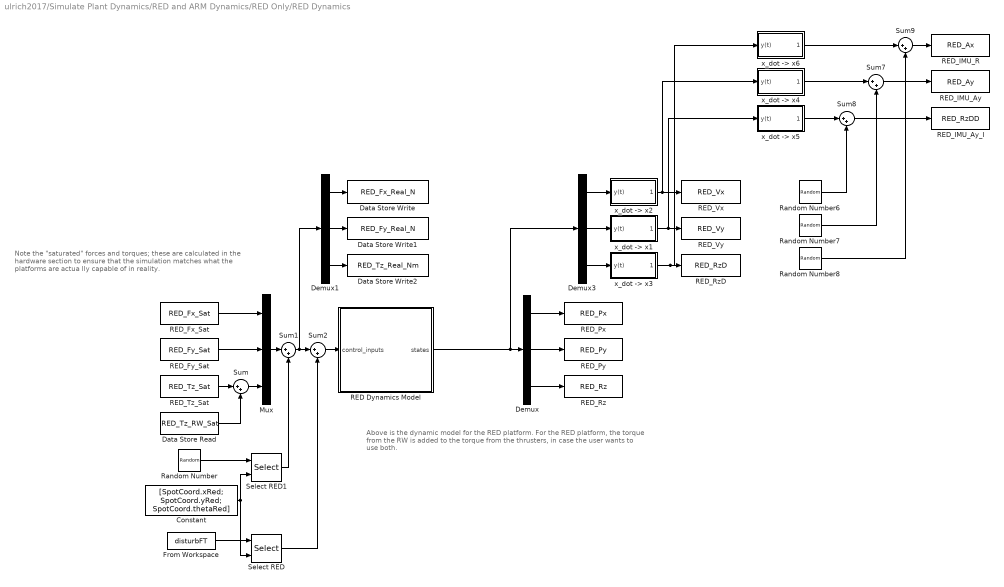
== system ulrich2017/Simulate Plant Dynamics/RED and ARM Dynamics/RED Only/RED Dynamics ==
  note: Above is the dynamic model for the RED
      | platform. For the RED platform, the torque from the RW is added to the torque from the thrusters, in case the user wants to use both.
  note: Note the "saturated" forces and torques; these are calculated in the hardware section to ensure that the simulation matches what the platforms are actua lly capable of in reality.
  Constant : Constant  Value=[SpotCoord.xRed; SpotCoord.yRed; SpotCoord.thetaRed]  VectorParams1D=off
  Data Store Read : DataStoreRead  DataStoreName=RED_Tz_RW_Sat  IndexOptions=Index vector (dialog)  Indices=1  OutputSizes=1
  Data Store Write : DataStoreWrite  DataStoreName=RED_Fx_Real_N  IndexOptions=Index vector (dialog)  Indices=1  OutputSizes=1
  Data Store Write1 : DataStoreWrite  DataStoreName=RED_Fy_Real_N  IndexOptions=Index vector (dialog)  Indices=1  OutputSizes=1
  Data Store Write2 : DataStoreWrite  DataStoreName=RED_Tz_Real_Nm  IndexOptions=Index vector (dialog)  Indices=1  OutputSizes=1
  Demux : Demux  Outputs=3
  Demux1 : Demux  Outputs=3
  Demux3 : Demux  Outputs=3
  From Workspace : FromWorkspace  VariableName=disturbFT
  Mux : Mux  Inputs=3
  RED Dynamics Model : Subsystem  SystemSampleTime=serverRate
  RED_Fx_Sat : DataStoreRead  DataStoreName=RED_Fx_Sat  IndexOptions=Index vector (dialog)  Indices=1  OutputSizes=1
  RED_Fy_Sat : DataStoreRead  DataStoreName=RED_Fy_Sat  IndexOptions=Index vector (dialog)  Indices=1  OutputSizes=1
  RED_IMU_Ay : DataStoreWrite  DataStoreName=RED_Ay  IndexOptions=Index vector (dialog)  Indices=1  OutputSizes=1
  RED_IMU_Ay_I : DataStoreWrite  DataStoreName=RED_RzDD  IndexOptions=Index vector (dialog)  Indices=1  OutputSizes=1
  RED_IMU_R : DataStoreWrite  DataStoreName=RED_Ax  IndexOptions=Index vector (dialog)  Indices=1  OutputSizes=1
  RED_Px : DataStoreWrite  DataStoreName=RED_Px  IndexOptions=Index vector (dialog)  Indices=1  OutputSizes=1
  RED_Py : DataStoreWrite  DataStoreName=RED_Py  IndexOptions=Index vector (dialog)  Indices=1  OutputSizes=1
  RED_Rz : DataStoreWrite  DataStoreName=RED_Rz  IndexOptions=Index vector (dialog)  Indices=1  OutputSizes=1
  RED_RzD : DataStoreWrite  DataStoreName=RED_RzD  IndexOptions=Index vector (dialog)  Indices=1  OutputSizes=1
  RED_Tz_Sat : DataStoreRead  DataStoreName=RED_Tz_Sat  IndexOptions=Index vector (dialog)  Indices=1  OutputSizes=1
  RED_Vx : DataStoreWrite  DataStoreName=RED_Vx  IndexOptions=Index vector (dialog)  Indices=1  OutputSizes=1
  RED_Vy : DataStoreWrite  DataStoreName=RED_Vy  IndexOptions=Index vector (dialog)  Indices=1  OutputSizes=1
  Random Number : RandomNumber  Mean=noiseFT.mean  Variance=noiseFT.var  Seed=noiseFT.seed
  Random Number6 : RandomNumber  Variance=1.5e-6
  Random Number7 : RandomNumber  Variance=1.5e-6
  Random Number8 : RandomNumber  Variance=1.5e-6
  Select RED : Selector  IndexOptions=Index vector (port)  Indices=[SpotCoord.xRed SpotCoord.yRed SpotCoord.thetaRed]  OutputSizes=1
  Select RED1 : Selector  IndexOptions=Index vector (port)  Indices=[SpotCoord.xRed SpotCoord.yRed SpotCoord.thetaRed]  OutputSizes=1
  Sum{,1..2,7..9} (6 alike) : Sum  Inputs=|++
  "x_dot -> x1" : Subsystem
  "x_dot -> x2" : Subsystem
  "x_dot -> x3" : Subsystem
  "x_dot -> x4" : Subsystem
  "x_dot -> x5" : Subsystem
  "x_dot -> x6" : Subsystem
  wires:
  Demux3/3 -> "x_dot -> x3"/1(y(t))
  "x_dot -> x2"/1(dy(t)/dt) -> "x_dot -> x4"/1(y(t)), RED_Vx/1
  Sum9/1 -> RED_IMU_R/1
  Demux3/2 -> "x_dot -> x1"/1(y(t))
  "x_dot -> x3"/1(dy(t)/dt) -> "x_dot -> x6"/1(y(t)), RED_RzD/1
  RED_Fy_Sat/1 -> Mux/2
  RED_Fx_Sat/1 -> Mux/1
  Demux/1 -> RED_Px/1
  Sum/1 -> Mux/3
  Demux3/1 -> "x_dot -> x2"/1(y(t))
  "x_dot -> x1"/1(dy(t)/dt) -> "x_dot -> x5"/1(y(t)), RED_Vy/1
  Data Store Read/1 -> Sum/2
  "x_dot -> x4"/1(dy(t)/dt) -> Sum7/1
  Random Number7/1 -> Sum7/2
  "x_dot -> x5"/1(dy(t)/dt) -> Sum8/1
  Random Number8/1 -> Sum9/2
  Demux/2 -> RED_Py/1
  Demux/3 -> RED_Rz/1
  RED_Tz_Sat/1 -> Sum/1
  Sum7/1 -> RED_IMU_Ay/1
  Sum8/1 -> RED_IMU_Ay_I/1
  Random Number6/1 -> Sum8/2
  RED Dynamics Model/1(states) -> Demux3/1, Demux/1
  "x_dot -> x6"/1(dy(t)/dt) -> Sum9/1
  From Workspace/1 -> Select RED/1
  Sum1/1 -> Demux1/1, Sum2/1
  Mux/1 -> Sum1/1
  Select RED/1 -> Sum2/2
  Select RED1/1 -> Sum1/2
  Constant/1 -> Select RED/2, Select RED1/2
  Random Number/1 -> Select RED1/1
  Demux1/3 -> Data Store Write2/1
  Demux1/1 -> Data Store Write/1
  Demux1/2 -> Data Store Write1/1
  Sum2/1 -> RED Dynamics Model/1(control_inputs)

== system ulrich2017/Thruster Control Code/Change BLACK Behavior/Calculate Thruster ON//OFF/Rotate Forces to Inertial ==
  "F_b " : Inport
  Rz : Inport  Port=2
  Create Rotation Matrix : MATLAB Function  TreatAsAtomicUnit=on
  Rotate F_b to F_I : Product  Multiplication=Matrix(*)
  F_I : Outport  VectorParamsAs1DForOutWhenUnconnected=off
  wires:
  "F_b "/1 -> Rotate F_b to F_I/2
  Rotate F_b to F_I/1 -> F_I/1
  Create Rotation Matrix/1(C_Ib) -> Rotate F_b to F_I/1
  Rz/1 -> Create Rotation Matrix/1(Rz)

== system ulrich2017/Thruster Control Code/Change BLACK Behavior/Calculate Thruster ON//OFF/pseudo-inverse ==
  H : Inport
  Product : Product  Multiplication=Matrix(*)
  Product1 : Product  Inputs=/  Multiplication=Matrix(*)
  Product2 : Product  Multiplication=Matrix(*)
  transpose : PermuteDimensions
  invH : Outport  VectorParamsAs1DForOutWhenUnconnected=off
  wires:
  Product2/1 -> invH/1
  transpose/1 -> Product/2, Product2/1
  Product/1 -> Product1/1
  H/1 -> Product/1, transpose/1
  Product1/1 -> Product2/2

== system ulrich2017/Thruster Control Code/Change BLACK Behavior/Calculate Thruster ON//OFF/pseudo-inverse3 ==
  H : Inport
  Product : Product  Multiplication=Matrix(*)
  Product1 : Product  Inputs=/  Multiplication=Matrix(*)
  Product2 : Product  Multiplication=Matrix(*)
  transpose : PermuteDimensions
  invH : Outport  VectorParamsAs1DForOutWhenUnconnected=off
  wires:
  Product2/1 -> invH/1
  transpose/1 -> Product/2, Product2/1
  Product/1 -> Product1/1
  H/1 -> Product/1, transpose/1
  Product1/1 -> Product2/2

== system ulrich2017/Thruster Control Code/Change BLUE Behavior/Calculate Thruster ON//OFF/Rotate Forces to Inertial ==
  "F_b " : Inport
  Rz : Inport  Port=2
  Create Rotation Matrix : MATLAB Function  TreatAsAtomicUnit=on
  Rotate F_b to F_I : Product  Multiplication=Matrix(*)
  F_I : Outport  VectorParamsAs1DForOutWhenUnconnected=off
  wires:
  "F_b "/1 -> Rotate F_b to F_I/2
  Rotate F_b to F_I/1 -> F_I/1
  Create Rotation Matrix/1(C_Ib) -> Rotate F_b to F_I/1
  Rz/1 -> Create Rotation Matrix/1(Rz)

== system ulrich2017/Thruster Control Code/Change BLUE Behavior/Calculate Thruster ON//OFF/pseudo-inverse ==
  H : Inport
  Product : Product  Multiplication=Matrix(*)
  Product1 : Product  Inputs=/  Multiplication=Matrix(*)
  Product2 : Product  Multiplication=Matrix(*)
  transpose : PermuteDimensions
  invH : Outport  VectorParamsAs1DForOutWhenUnconnected=off
  wires:
  Product2/1 -> invH/1
  transpose/1 -> Product/2, Product2/1
  Product/1 -> Product1/1
  H/1 -> Product/1, transpose/1
  Product1/1 -> Product2/2

== system ulrich2017/Thruster Control Code/Change BLUE Behavior/Calculate Thruster ON//OFF/pseudo-inverse2 ==
  H : Inport
  Product : Product  Multiplication=Matrix(*)
  Product1 : Product  Inputs=/  Multiplication=Matrix(*)
  Product2 : Product  Multiplication=Matrix(*)
  transpose : PermuteDimensions
  invH : Outport  VectorParamsAs1DForOutWhenUnconnected=off
  wires:
  Product2/1 -> invH/1
  transpose/1 -> Product/2, Product2/1
  Product/1 -> Product1/1
  H/1 -> Product/1, transpose/1
  Product1/1 -> Product2/2

== system ulrich2017/Thruster Control Code/Change RED Behavior/Calculate Thruster ON//OFF/If Action Subsystem ==
  In1 : Inport
  Action Port : ActionPort  ActionPortLabel=if(u1 == 4 | u1 == 5 | u1 == 10 | u1 == 11)
  Out1 : Outport
  wires:
  In1/1 -> Out1/1

== system ulrich2017/Thruster Control Code/Change RED Behavior/Calculate Thruster ON//OFF/If Action Subsystem1 ==
  In1 : Inport
  Action Port : ActionPort  ActionPortLabel=else
  Out1 : Outport
  wires:
  In1/1 -> Out1/1

== system ulrich2017/Thruster Control Code/Change RED Behavior/Calculate Thruster ON//OFF/If Action Subsystem2 ==
  In1 : Inport
  Action Port : ActionPort  ActionPortLabel=if(u1 == 4 | u1 == 5 | u1 == 10 | u1 == 11)
  Out1 : Outport
  wires:
  In1/1 -> Out1/1

== system ulrich2017/Thruster Control Code/Change RED Behavior/Calculate Thruster ON//OFF/If Action Subsystem3 ==
  H : Inport
  Action Port : ActionPort  ActionPortLabel=else
  Out1 : Outport
  wires:
  H/1 -> Out1/1

== system ulrich2017/Thruster Control Code/Change RED Behavior/Calculate Thruster ON//OFF/If Action Subsystem4 ==
  H : Inport
  Action Port : ActionPort  ActionPortLabel=if(u1 == 4 | u1 == 5 | u1 == 10 | u1 == 11)
  Out1 : Outport
  wires:
  H/1 -> Out1/1

== system ulrich2017/Thruster Control Code/Change RED Behavior/Calculate Thruster ON//OFF/If Action Subsystem5 ==
  In1 : Inport
  Action Port : ActionPort  ActionPortLabel=else
  Out1 : Outport
  wires:
  In1/1 -> Out1/1

== system ulrich2017/Thruster Control Code/Change RED Behavior/Calculate Thruster ON//OFF/Rotate Forces to Inertial ==
  "F_b " : Inport
  Rz : Inport  Port=2
  Create Rotation Matrix : MATLAB Function  TreatAsAtomicUnit=on
  Rotate F_b to F_I : Product  Multiplication=Matrix(*)
  F_I : Outport  VectorParamsAs1DForOutWhenUnconnected=off
  wires:
  "F_b "/1 -> Rotate F_b to F_I/2
  Rotate F_b to F_I/1 -> F_I/1
  Create Rotation Matrix/1(C_Ib) -> Rotate F_b to F_I/1
  Rz/1 -> Create Rotation Matrix/1(Rz)

== system ulrich2017/Thruster Control Code/Change RED Behavior/Calculate Thruster ON//OFF/pseudo-inverse ==
  H : Inport
  Product : Product  Multiplication=Matrix(*)
  Product1 : Product  Inputs=/  Multiplication=Matrix(*)
  Product2 : Product  Multiplication=Matrix(*)
  transpose : PermuteDimensions
  invH : Outport  VectorParamsAs1DForOutWhenUnconnected=off
  wires:
  Product2/1 -> invH/1
  transpose/1 -> Product/2, Product2/1
  Product/1 -> Product1/1
  H/1 -> Product/1, transpose/1
  Product1/1 -> Product2/2
